simulink model "sixuanyi_test"  (R2020a)
settings: Solver=ode45  StartTime=0.0  StopTime=inf  RelTol=1e-3
values from neighbouring files (symbols this model uses):
  P =     [Pdata.mat]
undefined symbols (not defined in the file or in its folder): plot_tracjectory
libraries: simulink x4
settings Model: Creator=陈帅  LastModifiedBy=陈帅

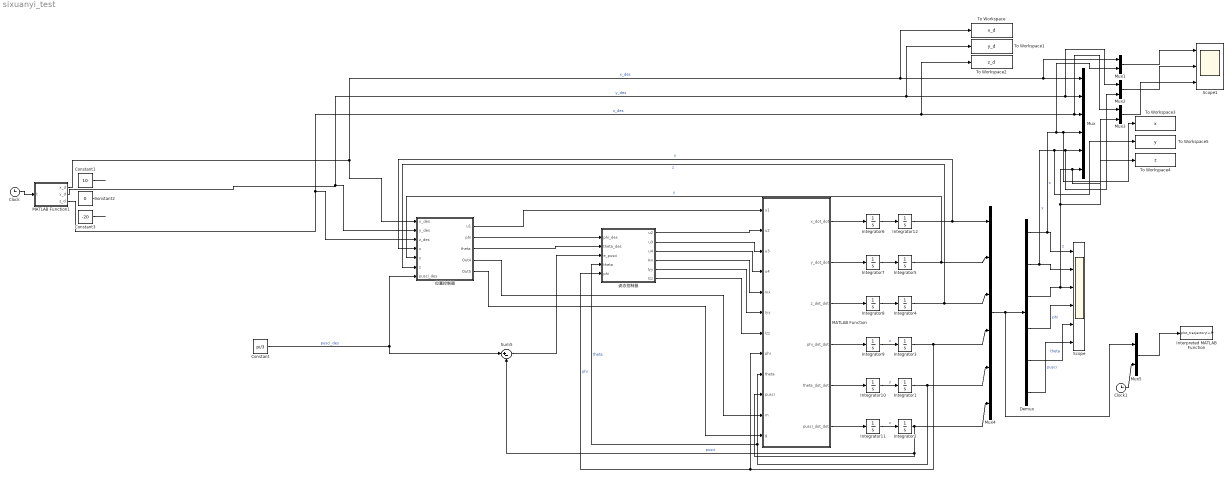
== system sixuanyi_test ==
  Clock : Clock
  Clock1 : Clock
  Constant : Constant  Value=pi/3
  Constant1 : Constant  Value=10
  Constant2 : Constant  Value=0
  Constant3 : Constant  Value=-20
  Demux : Demux  Outputs=6
  Integrator{1..12} (12 alike) : Integrator
  Interpreted MATLAB Function : MATLABFcn  MATLABFcn=plot_tracjectory(u,P)  OutputDimensions=0
  MATLAB Function : MATLAB Function  TreatAsAtomicUnit=on
  MATLAB Function1 : MATLAB Function  TreatAsAtomicUnit=on
  Mux : Mux  Inputs=6
  Mux{1..3,5} (4 alike) : Mux  Inputs=2
  Mux4 : Mux  Inputs=6
  Scope : Scope  NumInputPorts=6
  Scope1 : Scope  NumInputPorts=3
  Sum5 : Sum  Inputs=|+-
  To Workspace : ToWorkspace  VariableName=x_d  SampleTime=-1
      settings: Save2DSignal=2-D array (concatenate along first dimension)
  To Workspace1 : ToWorkspace  VariableName=y_d  SampleTime=-1
      settings: Save2DSignal=2-D array (concatenate along first dimension)
  To Workspace2 : ToWorkspace  VariableName=z_d  SampleTime=-1
      settings: Save2DSignal=2-D array (concatenate along first dimension)
  To Workspace3 : ToWorkspace  VariableName=x  SampleTime=-1
      settings: Save2DSignal=2-D array (concatenate along first dimension)
  To Workspace4 : ToWorkspace  VariableName=z  SampleTime=-1
      settings: Save2DSignal=2-D array (concatenate along first dimension)
  To Workspace5 : ToWorkspace  VariableName=y  SampleTime=-1
      settings: Save2DSignal=2-D array (concatenate along first dimension)
  位置控制器 : Subsystem
  姿态控制器 : Subsystem
  wires:
  Integrator9/1 -> Integrator3/1  "x"
  Integrator10/1 -> Integrator1/1  "y"
  Integrator11/1 -> Integrator2/1  "z"
  MATLAB Function/4(phi_dot_dot) -> Integrator9/1
  MATLAB Function/5(theta_dot_dot) -> Integrator10/1
  MATLAB Function/6(pusci_dot_dot) -> Integrator11/1
  Integrator3/1 -> 姿态控制器/5(phi), MATLAB Function/8(phi), Mux4/4  "phi"
  Integrator1/1 -> Mux4/5, 姿态控制器/4(theta), MATLAB Function/9(theta)  "theta"
  Constant/1 -> Sum5/1, 位置控制器/7(pusci_des)  "pusci_des"
  Integrator2/1 -> MATLAB Function/10(pusci), Sum5/2, Mux4/6  "pusci"
  MATLAB Function/3(z_dot_dot) -> Integrator8/1
  Integrator8/1 -> Integrator4/1
  MATLAB Function/2(y_dot_dot) -> Integrator7/1
  MATLAB Function/1(x_dot_dot) -> Integrator6/1
  Integrator6/1 -> Integrator12/1
  Integrator4/1 -> 位置控制器/6(z), Mux4/3  "z"
  Integrator7/1 -> Integrator5/1
  Integrator12/1 -> 位置控制器/4(x), Mux4/1  "x"
  Integrator5/1 -> 位置控制器/5(y), Mux4/2  "y"
  Mux4/1 -> Mux5/1, Demux/1
  Demux/1 -> Mux1/2, To Workspace3/1, Mux/4, Scope/1  "x"
  Demux/2 -> To Workspace5/1, Mux2/2, Mux/5, Scope/2  "y"
  Demux/3 -> To Workspace4/1, Mux3/2, Mux/6, Scope/3  "z"
  Demux/4 -> Scope/4  "phi"
  Demux/5 -> Scope/5  "theta"
  Demux/6 -> Scope/6  "pusci"
  Sum5/1 -> 姿态控制器/3(e_pusci)
  姿态控制器/1(u2) -> MATLAB Function/2(u2)
  姿态控制器/2(u3) -> MATLAB Function/3(u3)
  姿态控制器/3(u4) -> MATLAB Function/4(u4)
  姿态控制器/4(Ixx) -> MATLAB Function/5(Ixx)
  姿态控制器/5(Iyy) -> MATLAB Function/6(Iyy)
  姿态控制器/6(Izz) -> MATLAB Function/7(Izz)
  MATLAB Function1/1(x_d) -> 位置控制器/1(x_des), To Workspace/1, Mux1/1, Mux/1  "x_des"
  MATLAB Function1/2(y_d) -> To Workspace1/1, Mux2/1, Mux/2, 位置控制器/2(y_des)  "y_des"
  MATLAB Function1/3(z_d) -> To Workspace2/1, Mux3/1, Mux/3, 位置控制器/3(z_des)  "z_des"
  位置控制器/1(u1) -> MATLAB Function/1(u1)
  位置控制器/2(phi) -> 姿态控制器/1(phi_des)
  位置控制器/3(theta) -> 姿态控制器/2(theta_des)
  位置控制器/4(Out4) -> MATLAB Function/11(m)
  位置控制器/5(Out5) -> MATLAB Function/12(g)
  Mux1/1 -> Scope1/1
  Mux2/1 -> Scope1/2
  Mux3/1 -> Scope1/3
  Mux5/1 -> Interpreted MATLAB Function/1
  Clock1/1 -> Mux5/2
  Constant1/1 -> ?
  Constant2/1 -> ?
  Constant3/1 -> ?
  Clock/1 -> MATLAB Function1/1(t)

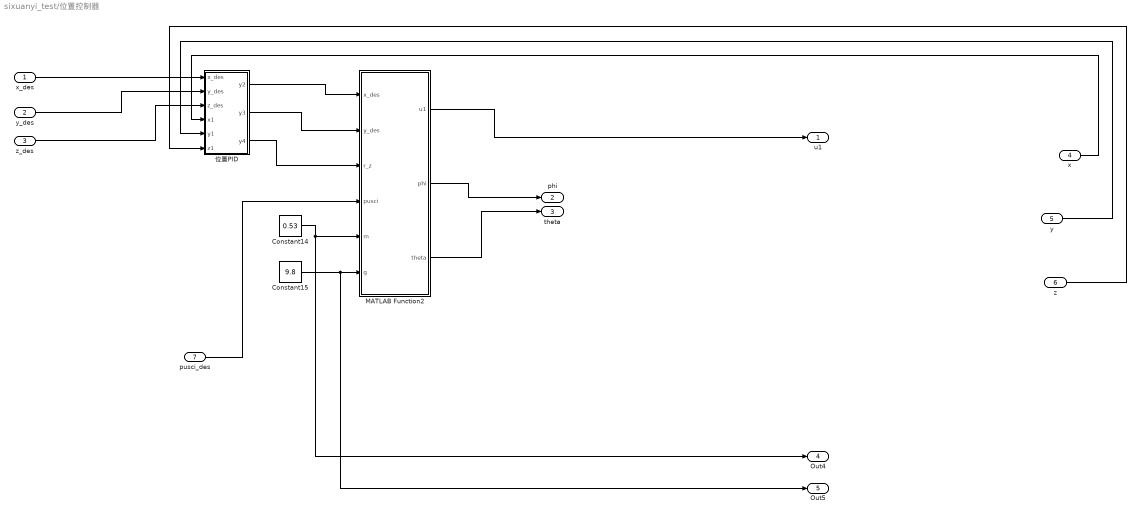
== system sixuanyi_test/位置控制器 ==
  x_des : Inport
  y_des : Inport  Port=2
  z_des : Inport  Port=3
  x : Inport  Port=4
  y : Inport  Port=5
  z : Inport  Port=6
  pusci_des : Inport  Port=7
  Constant14 : Constant  Value=0.53
  Constant15 : Constant  Value=9.8
  MATLAB Function2 : MATLAB Function  TreatAsAtomicUnit=on
  位置PID : Subsystem
  u1 : Outport
  phi : Outport  Port=2
  theta : Outport  Port=3
  Out4 : Outport  Port=4
  Out5 : Outport  Port=5
  wires:
  Constant14/1 -> Out4/1, MATLAB Function2/5(m)
  位置PID/1(y2) -> MATLAB Function2/1(x_des)
  y/1 -> 位置PID/5(y1)
  MATLAB Function2/3(theta) -> theta/1
  pusci_des/1 -> MATLAB Function2/4(pusci)
  位置PID/2(y3) -> MATLAB Function2/2(y_des)
  y_des/1 -> 位置PID/2(y_des)
  Constant15/1 -> Out5/1, MATLAB Function2/6(g)
  MATLAB Function2/1(u1) -> u1/1
  x_des/1 -> 位置PID/1(x_des)
  位置PID/3(y4) -> MATLAB Function2/3(r_z)
  x/1 -> 位置PID/4(x1)
  MATLAB Function2/2(phi) -> phi/1
  z/1 -> 位置PID/6(z1)
  z_des/1 -> 位置PID/3(z_des)

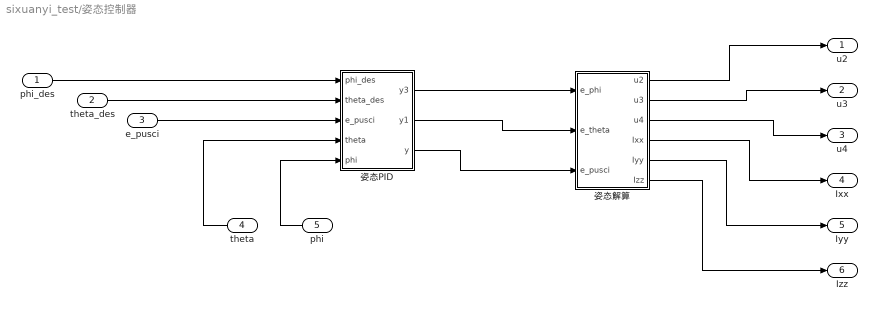
== system sixuanyi_test/姿态控制器 ==
  phi_des : Inport
  theta_des : Inport  Port=2
  e_pusci : Inport  Port=3
  theta : Inport  Port=4
  phi : Inport  Port=5
  姿态PID : Subsystem
  姿态解算 : Subsystem
  u2 : Outport
  u3 : Outport  Port=2
  u4 : Outport  Port=3
  Ixx : Outport  Port=4
  Iyy : Outport  Port=5
  Izz : Outport  Port=6
  wires:
  姿态解算/3(u4) -> u4/1
  姿态PID/2(y1) -> 姿态解算/2(e_theta)
  姿态解算/5(Iyy) -> Iyy/1
  姿态解算/6(Izz) -> Izz/1
  姿态PID/3(y) -> 姿态解算/3(e_pusci)
  姿态PID/1(y3) -> 姿态解算/1(e_phi)
  phi_des/1 -> 姿态PID/1(phi_des)
  e_pusci/1 -> 姿态PID/3(e_pusci)
  姿态解算/4(Ixx) -> Ixx/1
  姿态解算/2(u3) -> u3/1
  姿态解算/1(u2) -> u2/1
  theta_des/1 -> 姿态PID/2(theta_des)
  phi/1 -> 姿态PID/5(phi)
  theta/1 -> 姿态PID/4(theta)

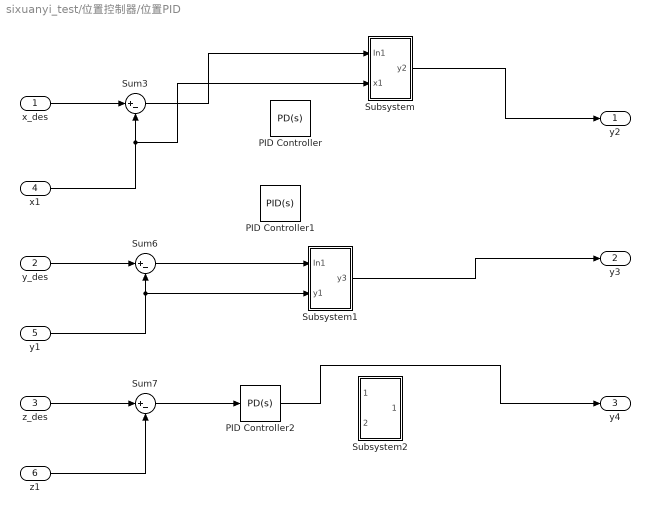
== system sixuanyi_test/位置控制器/位置PID ==
  x_des : Inport
  y_des : Inport  Port=2
  z_des : Inport  Port=3
  x1 : Inport  Port=4
  y1 : Inport  Port=5
  z1 : Inport  Port=6
  PID Controller : simulink/Continuous/PID Controller  Controller=PD  Form=Parallel  TimeDomain=Continuous-time  UseExternalTs=off  SampleTime=-1  IntegratorMethod=Forward Euler  FilterMethod=Forward Euler  ControllerParametersSource=internal  P=0.0127137328942064  I=6.25628714194927e-05  D=0.574050981950461  UseFilter=on  N=96.3969564252271  TunerSelectOption=Transfer Function Based (PID Tuner App)  InitialConditionSource=internal  InitialConditionForIntegrator=0  InitialConditionForFilter=0  DifferentiatorICPrevScaledInput=0  ExternalReset=none  TrackingMode=off  Kt=1  LimitOutput=off  UpperSaturationLimit=inf  LowerSaturationLimit=-inf  LinearizeAsGain=on  AntiWindupMode=none  Kb=1  POutMin=[]  POutMax=[]  IOutMin=[]  IOutMax=[]  DOutMin=[]  DOutMax=[]  NOutMin=[]  NOutMax=[]  SumOutMin=[]  SumOutMax=[]  SaturationOutMin=[]  SaturationOutMax=[]  PParamMin=[]  PParamMax=[]  IParamMin=[]  IParamMax=[]  DParamMin=[]  DParamMax=[]  NParamMin=[]  NParamMax=[]  KbParamMin=[]  KbParamMax=[]  KtParamMin=[]  KtParamMax=[]  KbOutMin=[]  KbOutMax=[]  KtOutMin=[]  KtOutMax=[]  IntegratorOutMin=[]  IntegratorOutMax=[]  FilterOutMin=[]  FilterOutMax=[]  SumI1OutMin=[]  SumI1OutMax=[]  SumI2OutMin=[]  SumI2OutMax=[]  SumI3OutMin=[]  SumI3OutMax=[]  SumI4OutMin=[]  SumI4OutMax=[]  SumDOutMin=[]  SumDOutMax=[]  DifferentiatorOutMin=[]  DifferentiatorOutMax=[]  FilterDiffOutCoefMin=[]  FilterDiffOutCoefMax=[]  ReciprocalOutMin=[]  ReciprocalOutMax=[]  SumDenOutMin=[]  SumDenOutMax=[]  SumNumOutMin=[]  SumNumOutMax=[]  DivideOutMin=[]  DivideOutMax=[]  UdiffTsProdOutMin=[]  UdiffTsProdOutMax=[]  NTsProdOutMin=[]  NTsProdOutMax=[]  UintegralTsProdOutMin=[]  UintegralTsProdOutMax=[]  UngainTsProdOutMin=[]  UngainTsProdOutMax=[]  IntegratorContinuousStateAttributes=''  IntegratorStateMustResolveToSignalObject=off  IntegratorRTWStateStorageClass=Auto  FilterContinuousStateAttributes=''  FilterStateMustResolveToSignalObject=off  FilterRTWStateStorageClass=Auto  ParallelPVariant=InternalParameters  IdealPVariant=Disabled  IVariant=Disabled  DVariant=InternalParameters  IntegratorVariant=Disabled  SatVariant=Disabled  AWVariant=Disabled  PCopyVariant=Disabled  TRVariant=Disabled  FdbkBlocksVariant=Forward  IdealPFdbkVariant=Disabled  SatFdbkVariant=Disabled  DerivativeFilterVariant=ContFilter  NVariant=InternalParameters  NCopyVariant=Disabled  FilterICVariant=InternalICsFilter  IntegratorICVariant=Disabled  ExternalResetVariant=Disabled  TRSumVariant=Passthrough  SumFdbkVariant=Disabled  SumVariant=Sum_PD  TsampFilterVariant=InternalTs  TsampNgainVariant=Passthrough  TsampIntegralVariant=Disabled_SignalSpec
  PID Controller1 : simulink/Continuous/PID Controller  Controller=PID  Form=Parallel  TimeDomain=Continuous-time  UseExternalTs=off  SampleTime=-1  IntegratorMethod=Forward Euler  FilterMethod=Forward Euler  ControllerParametersSource=internal  P=0.0236681294333178  I=0  D=0.611835999148078  UseFilter=on  N=102.587789590808  TunerSelectOption=Transfer Function Based (PID Tuner App)  InitialConditionSource=internal  InitialConditionForIntegrator=0  InitialConditionForFilter=0  DifferentiatorICPrevScaledInput=0  ExternalReset=none  TrackingMode=off  Kt=1  LimitOutput=off  UpperSaturationLimit=inf  LowerSaturationLimit=-inf  LinearizeAsGain=on  AntiWindupMode=none  Kb=1  POutMin=[]  POutMax=[]  IOutMin=[]  IOutMax=[]  DOutMin=[]  DOutMax=[]  NOutMin=[]  NOutMax=[]  SumOutMin=[]  SumOutMax=[]  SaturationOutMin=[]  SaturationOutMax=[]  PParamMin=[]  PParamMax=[]  IParamMin=[]  IParamMax=[]  DParamMin=[]  DParamMax=[]  NParamMin=[]  NParamMax=[]  KbParamMin=[]  KbParamMax=[]  KtParamMin=[]  KtParamMax=[]  KbOutMin=[]  KbOutMax=[]  KtOutMin=[]  KtOutMax=[]  IntegratorOutMin=[]  IntegratorOutMax=[]  FilterOutMin=[]  FilterOutMax=[]  SumI1OutMin=[]  SumI1OutMax=[]  SumI2OutMin=[]  SumI2OutMax=[]  SumI3OutMin=[]  SumI3OutMax=[]  SumI4OutMin=[]  SumI4OutMax=[]  SumDOutMin=[]  SumDOutMax=[]  DifferentiatorOutMin=[]  DifferentiatorOutMax=[]  FilterDiffOutCoefMin=[]  FilterDiffOutCoefMax=[]  ReciprocalOutMin=[]  ReciprocalOutMax=[]  SumDenOutMin=[]  SumDenOutMax=[]  SumNumOutMin=[]  SumNumOutMax=[]  DivideOutMin=[]  DivideOutMax=[]  UdiffTsProdOutMin=[]  UdiffTsProdOutMax=[]  NTsProdOutMin=[]  NTsProdOutMax=[]  UintegralTsProdOutMin=[]  UintegralTsProdOutMax=[]  UngainTsProdOutMin=[]  UngainTsProdOutMax=[]  IntegratorContinuousStateAttributes=''  IntegratorStateMustResolveToSignalObject=off  IntegratorRTWStateStorageClass=Auto  FilterContinuousStateAttributes=''  FilterStateMustResolveToSignalObject=off  FilterRTWStateStorageClass=Auto  ParallelPVariant=InternalParameters  IdealPVariant=Disabled  IVariant=InternalParameters  DVariant=InternalParameters  IntegratorVariant=Continuous  SatVariant=Disabled  AWVariant=Passthrough  PCopyVariant=Disabled  TRVariant=Disabled  FdbkBlocksVariant=Forward  IdealPFdbkVariant=Disabled  SatFdbkVariant=Disabled  DerivativeFilterVariant=ContFilter  NVariant=InternalParameters  NCopyVariant=Disabled  FilterICVariant=InternalICsFilter  IntegratorICVariant=InternalICs  ExternalResetVariant=Disabled  TRSumVariant=Passthrough  SumFdbkVariant=Disabled  SumVariant=Sum_PID  TsampFilterVariant=InternalTs  TsampNgainVariant=Passthrough  TsampIntegralVariant=Passthrough
  PID Controller2 : simulink/Continuous/PID Controller  Controller=PD  Form=Parallel  TimeDomain=Continuous-time  UseExternalTs=off  SampleTime=-1  IntegratorMethod=Forward Euler  FilterMethod=Forward Euler  ControllerParametersSource=internal  P=1.56802475831862  I=1  D=8.31416999663837  UseFilter=on  N=950.562907073993  TunerSelectOption=Transfer Function Based (PID Tuner App)  InitialConditionSource=internal  InitialConditionForIntegrator=0  InitialConditionForFilter=0  DifferentiatorICPrevScaledInput=0  ExternalReset=none  TrackingMode=off  Kt=1  LimitOutput=off  UpperSaturationLimit=inf  LowerSaturationLimit=-inf  LinearizeAsGain=on  AntiWindupMode=none  Kb=1  POutMin=[]  POutMax=[]  IOutMin=[]  IOutMax=[]  DOutMin=[]  DOutMax=[]  NOutMin=[]  NOutMax=[]  SumOutMin=[]  SumOutMax=[]  SaturationOutMin=[]  SaturationOutMax=[]  PParamMin=[]  PParamMax=[]  IParamMin=[]  IParamMax=[]  DParamMin=[]  DParamMax=[]  NParamMin=[]  NParamMax=[]  KbParamMin=[]  KbParamMax=[]  KtParamMin=[]  KtParamMax=[]  KbOutMin=[]  KbOutMax=[]  KtOutMin=[]  KtOutMax=[]  IntegratorOutMin=[]  IntegratorOutMax=[]  FilterOutMin=[]  FilterOutMax=[]  SumI1OutMin=[]  SumI1OutMax=[]  SumI2OutMin=[]  SumI2OutMax=[]  SumI3OutMin=[]  SumI3OutMax=[]  SumI4OutMin=[]  SumI4OutMax=[]  SumDOutMin=[]  SumDOutMax=[]  DifferentiatorOutMin=[]  DifferentiatorOutMax=[]  FilterDiffOutCoefMin=[]  FilterDiffOutCoefMax=[]  ReciprocalOutMin=[]  ReciprocalOutMax=[]  SumDenOutMin=[]  SumDenOutMax=[]  SumNumOutMin=[]  SumNumOutMax=[]  DivideOutMin=[]  DivideOutMax=[]  UdiffTsProdOutMin=[]  UdiffTsProdOutMax=[]  NTsProdOutMin=[]  NTsProdOutMax=[]  UintegralTsProdOutMin=[]  UintegralTsProdOutMax=[]  UngainTsProdOutMin=[]  UngainTsProdOutMax=[]  IntegratorContinuousStateAttributes=''  IntegratorStateMustResolveToSignalObject=off  IntegratorRTWStateStorageClass=Auto  FilterContinuousStateAttributes=''  FilterStateMustResolveToSignalObject=off  FilterRTWStateStorageClass=Auto  ParallelPVariant=InternalParameters  IdealPVariant=Disabled  IVariant=Disabled  DVariant=InternalParameters  IntegratorVariant=Disabled  SatVariant=Disabled  AWVariant=Disabled  PCopyVariant=Disabled  TRVariant=Disabled  FdbkBlocksVariant=Forward  IdealPFdbkVariant=Disabled  SatFdbkVariant=Disabled  DerivativeFilterVariant=ContFilter  NVariant=InternalParameters  NCopyVariant=Disabled  FilterICVariant=InternalICsFilter  IntegratorICVariant=Disabled  ExternalResetVariant=Disabled  TRSumVariant=Passthrough  SumFdbkVariant=Disabled  SumVariant=Sum_PD  TsampFilterVariant=InternalTs  TsampNgainVariant=Passthrough  TsampIntegralVariant=Disabled_SignalSpec
  Subsystem : Subsystem
  Subsystem1 : Subsystem
  Subsystem2 : Subsystem
  Sum3 : Sum  Inputs=|+-
  Sum6 : Sum  Inputs=|+-
  Sum7 : Sum  Inputs=|+-
  y2 : Outport
  y3 : Outport  Port=2
  y4 : Outport  Port=3
  wires:
  z_des/1 -> Sum7/1
  y_des/1 -> Sum6/1
  x1/1 -> Subsystem/2(x1), Sum3/2
  x_des/1 -> Sum3/1
  y1/1 -> Subsystem1/2(y1), Sum6/2
  z1/1 -> Sum7/2
  Sum7/1 -> PID Controller2/1
  PID Controller2/1 -> y4/1
  Subsystem1/1(y3) -> y3/1
  Sum6/1 -> Subsystem1/1(In1)
  Sum3/1 -> Subsystem/1(In1)
  Subsystem/1(y2) -> y2/1

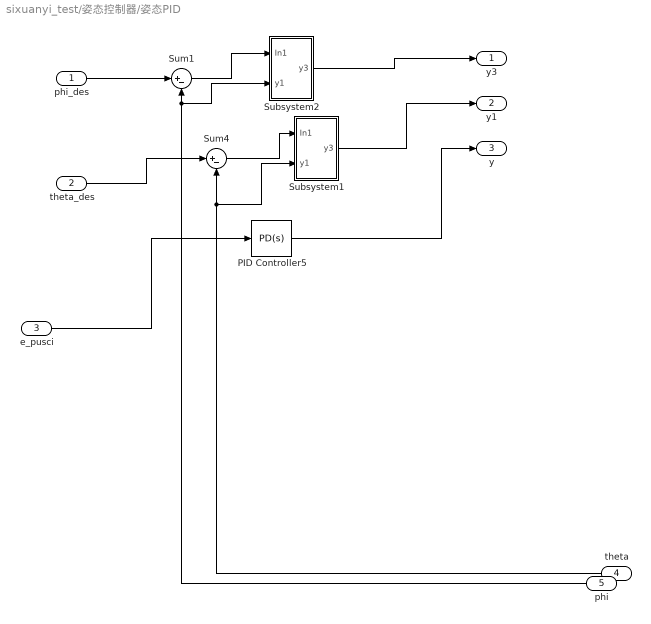
== system sixuanyi_test/姿态控制器/姿态PID ==
  phi_des : Inport
  theta_des : Inport  Port=2
  e_pusci : Inport  Port=3
  theta : Inport  Port=4
  phi : Inport  Port=5
  PID Controller5 : simulink/Continuous/PID Controller  Controller=PD  Form=Parallel  TimeDomain=Continuous-time  UseExternalTs=off  SampleTime=-1  IntegratorMethod=Forward Euler  FilterMethod=Forward Euler  ControllerParametersSource=internal  P=5.26569653292964  I=0  D=4.89151407738421  UseFilter=on  N=572.770791824144  TunerSelectOption=Transfer Function Based (PID Tuner App)  InitialConditionSource=internal  InitialConditionForIntegrator=0  InitialConditionForFilter=0  DifferentiatorICPrevScaledInput=0  ExternalReset=none  TrackingMode=off  Kt=1  LimitOutput=off  UpperSaturationLimit=inf  LowerSaturationLimit=-inf  LinearizeAsGain=on  AntiWindupMode=none  Kb=1  POutMin=[]  POutMax=[]  IOutMin=[]  IOutMax=[]  DOutMin=[]  DOutMax=[]  NOutMin=[]  NOutMax=[]  SumOutMin=[]  SumOutMax=[]  SaturationOutMin=[]  SaturationOutMax=[]  PParamMin=[]  PParamMax=[]  IParamMin=[]  IParamMax=[]  DParamMin=[]  DParamMax=[]  NParamMin=[]  NParamMax=[]  KbParamMin=[]  KbParamMax=[]  KtParamMin=[]  KtParamMax=[]  KbOutMin=[]  KbOutMax=[]  KtOutMin=[]  KtOutMax=[]  IntegratorOutMin=[]  IntegratorOutMax=[]  FilterOutMin=[]  FilterOutMax=[]  SumI1OutMin=[]  SumI1OutMax=[]  SumI2OutMin=[]  SumI2OutMax=[]  SumI3OutMin=[]  SumI3OutMax=[]  SumI4OutMin=[]  SumI4OutMax=[]  SumDOutMin=[]  SumDOutMax=[]  DifferentiatorOutMin=[]  DifferentiatorOutMax=[]  FilterDiffOutCoefMin=[]  FilterDiffOutCoefMax=[]  ReciprocalOutMin=[]  ReciprocalOutMax=[]  SumDenOutMin=[]  SumDenOutMax=[]  SumNumOutMin=[]  SumNumOutMax=[]  DivideOutMin=[]  DivideOutMax=[]  UdiffTsProdOutMin=[]  UdiffTsProdOutMax=[]  NTsProdOutMin=[]  NTsProdOutMax=[]  UintegralTsProdOutMin=[]  UintegralTsProdOutMax=[]  UngainTsProdOutMin=[]  UngainTsProdOutMax=[]  IntegratorContinuousStateAttributes=''  IntegratorStateMustResolveToSignalObject=off  IntegratorRTWStateStorageClass=Auto  FilterContinuousStateAttributes=''  FilterStateMustResolveToSignalObject=off  FilterRTWStateStorageClass=Auto  ParallelPVariant=InternalParameters  IdealPVariant=Disabled  IVariant=Disabled  DVariant=InternalParameters  IntegratorVariant=Disabled  SatVariant=Disabled  AWVariant=Disabled  PCopyVariant=Disabled  TRVariant=Disabled  FdbkBlocksVariant=Forward  IdealPFdbkVariant=Disabled  SatFdbkVariant=Disabled  DerivativeFilterVariant=ContFilter  NVariant=InternalParameters  NCopyVariant=Disabled  FilterICVariant=InternalICsFilter  IntegratorICVariant=Disabled  ExternalResetVariant=Disabled  TRSumVariant=Passthrough  SumFdbkVariant=Disabled  SumVariant=Sum_PD  TsampFilterVariant=InternalTs  TsampNgainVariant=Passthrough  TsampIntegralVariant=Disabled_SignalSpec
  Subsystem1 : Subsystem
  Subsystem2 : Subsystem
  Sum1 : Sum  Inputs=|+-
  Sum4 : Sum  Inputs=|+-
  y3 : Outport
  y1 : Outport  Port=2
  y : Outport  Port=3
  wires:
  Sum4/1 -> Subsystem1/1(In1)
  theta_des/1 -> Sum4/1
  phi_des/1 -> Sum1/1
  theta/1 -> Subsystem1/2(y1), Sum4/2
  phi/1 -> Subsystem2/2(y1), Sum1/2
  PID Controller5/1 -> y/1
  e_pusci/1 -> PID Controller5/1
  Subsystem2/1(y3) -> y3/1
  Sum1/1 -> Subsystem2/1(In1)
  Subsystem1/1(y3) -> y1/1

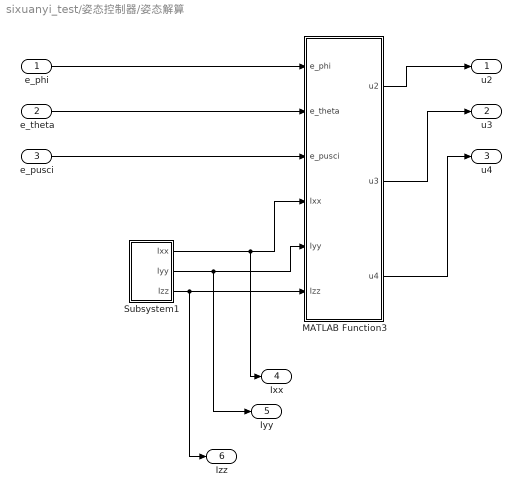
== system sixuanyi_test/姿态控制器/姿态解算 ==
  e_phi : Inport
  e_theta : Inport  Port=2
  e_pusci : Inport  Port=3
  MATLAB Function3 : MATLAB Function  TreatAsAtomicUnit=on
  Subsystem1 : Subsystem
  u2 : Outport
  u3 : Outport  Port=2
  u4 : Outport  Port=3
  Ixx : Outport  Port=4
  Iyy : Outport  Port=5
  Izz : Outport  Port=6
  wires:
  e_theta/1 -> MATLAB Function3/2(e_theta)
  Subsystem1/2(Iyy) -> MATLAB Function3/5(Iyy), Iyy/1
  Subsystem1/1(Ixx) -> MATLAB Function3/4(Ixx), Ixx/1
  e_pusci/1 -> MATLAB Function3/3(e_pusci)
  Subsystem1/3(Izz) -> MATLAB Function3/6(Izz), Izz/1
  MATLAB Function3/1(u2) -> u2/1
  e_phi/1 -> MATLAB Function3/1(e_phi)
  MATLAB Function3/2(u3) -> u3/1
  MATLAB Function3/3(u4) -> u4/1

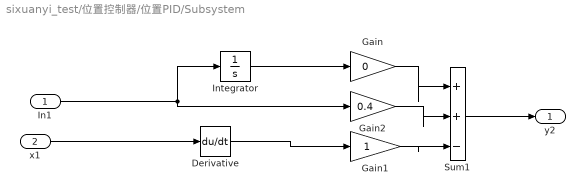
== system sixuanyi_test/位置控制器/位置PID/Subsystem ==
  In1 : Inport
  x1 : Inport  Port=2
  Derivative : Derivative
  Gain : Gain  Gain=0
  Gain1 : Gain
  Gain2 : Gain  Gain=0.4
  Integrator : Integrator
  Sum1 : Sum  Inputs=|++-
  y2 : Outport
  wires:
  In1/1 -> Gain2/1, Integrator/1
  Gain/1 -> Sum1/1
  Derivative/1 -> Gain1/1
  Gain1/1 -> Sum1/3
  Integrator/1 -> Gain/1
  Sum1/1 -> y2/1
  Gain2/1 -> Sum1/2
  x1/1 -> Derivative/1

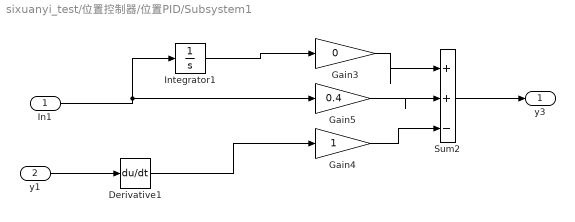
== system sixuanyi_test/位置控制器/位置PID/Subsystem1 ==
  In1 : Inport
  y1 : Inport  Port=2
  Derivative1 : Derivative
  Gain3 : Gain  Gain=0
  Gain4 : Gain
  Gain5 : Gain  Gain=0.4
  Integrator1 : Integrator
  Sum2 : Sum  Inputs=|++-
  y3 : Outport
  wires:
  Integrator1/1 -> Gain3/1
  In1/1 -> Integrator1/1, Gain5/1
  Gain4/1 -> Sum2/3
  Derivative1/1 -> Gain4/1
  Gain3/1 -> Sum2/1
  y1/1 -> Derivative1/1
  Gain5/1 -> Sum2/2
  Sum2/1 -> y3/1

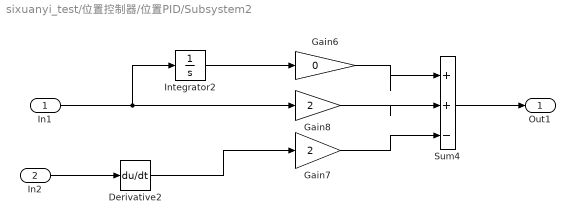
== system sixuanyi_test/位置控制器/位置PID/Subsystem2 ==
  In1 : Inport
  In2 : Inport  Port=2
  Derivative2 : Derivative
  Gain6 : Gain  Gain=0
  Gain7 : Gain  Gain=2
  Gain8 : Gain  Gain=2
  Integrator2 : Integrator
  Sum4 : Sum  Inputs=|++-
  Out1 : Outport
  wires:
  In2/1 -> Derivative2/1
  Integrator2/1 -> Gain6/1
  Gain6/1 -> Sum4/1
  Derivative2/1 -> Gain7/1
  Gain8/1 -> Sum4/2
  Gain7/1 -> Sum4/3
  In1/1 -> Integrator2/1, Gain8/1
  Sum4/1 -> Out1/1

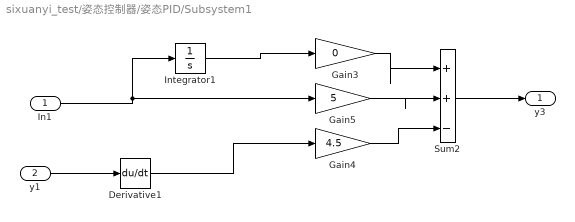
== system sixuanyi_test/姿态控制器/姿态PID/Subsystem1 ==
  In1 : Inport
  y1 : Inport  Port=2
  Derivative1 : Derivative
  Gain3 : Gain  Gain=0
  Gain4 : Gain  Gain=4.5
  Gain5 : Gain  Gain=5
  Integrator1 : Integrator
  Sum2 : Sum  Inputs=|++-
  y3 : Outport
  wires:
  Integrator1/1 -> Gain3/1
  In1/1 -> Integrator1/1, Gain5/1
  Gain4/1 -> Sum2/3
  Derivative1/1 -> Gain4/1
  Gain3/1 -> Sum2/1
  y1/1 -> Derivative1/1
  Gain5/1 -> Sum2/2
  Sum2/1 -> y3/1

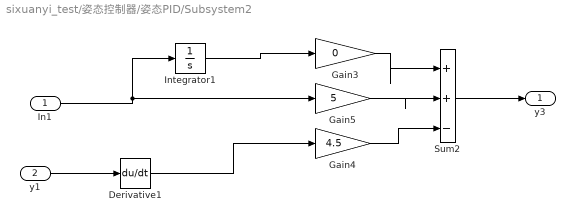
== system sixuanyi_test/姿态控制器/姿态PID/Subsystem2 ==
  In1 : Inport
  y1 : Inport  Port=2
  Derivative1 : Derivative
  Gain3 : Gain  Gain=0
  Gain4 : Gain  Gain=4.5
  Gain5 : Gain  Gain=5
  Integrator1 : Integrator
  Sum2 : Sum  Inputs=|++-
  y3 : Outport
  wires:
  Sum2/1 -> y3/1
  Gain5/1 -> Sum2/2
  y1/1 -> Derivative1/1
  Gain3/1 -> Sum2/1
  Derivative1/1 -> Gain4/1
  Gain4/1 -> Sum2/3
  In1/1 -> Gain5/1, Integrator1/1
  Integrator1/1 -> Gain3/1

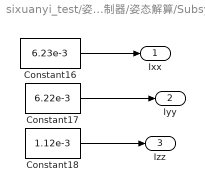
== system sixuanyi_test/姿态控制器/姿态解算/Subsystem1 ==
  Constant16 : Constant  Value=6.23e-3
  Constant17 : Constant  Value=6.22e-3
  Constant18 : Constant  Value=1.12e-3
  Ixx : Outport
  Iyy : Outport  Port=2
  Izz : Outport  Port=3
  wires:
  Constant18/1 -> Izz/1
  Constant16/1 -> Ixx/1
  Constant17/1 -> Iyy/1

== matlab function sixuanyi_test/MATLAB Function1 ==
  data: t input; x_d output; y_d output; z_d output
function [x_d,y_d,z_d]= fcn(t)
x_d=cos(t/2);
y_d=sin(t/2);
z_d=-0.2*t;
end

== matlab function sixuanyi_test/MATLAB Function ==
  data: u1 input; u2 input; u3 input; u4 input; x_dot_dot output; y_dot_dot output; z_dot_dot output; phi_dot_dot output; theta_dot_dot output; pusci_dot_dot output; Ixx input; Iyy input; Izz input; phi input; theta input; pusci input; m input; g input
function [x_dot_dot,y_dot_dot,z_dot_dot,phi_dot_dot,theta_dot_dot,pusci_dot_dot]=dynamic(u1,u2,u3,u4,Ixx,Iyy,Izz,phi,theta,pusci,m,g)

x_dot_dot=-u1/m*(sin(pusci)*phi+cos(pusci)*theta);
y_dot_dot=-u1/m*(-cos(pusci)*phi+theta*sin(pusci));
z_dot_dot=g-u1/m*cos(theta)*cos(phi);

phi_dot_dot=u2/Ixx;
theta_dot_dot=u3/Iyy;
pusci_dot_dot=u4/Izz;

end

== matlab function sixuanyi_test/位置控制器/MATLAB Function2 ==
  data: u1 output; x_des input; y_des input; r_z input; pusci input; m input; g input; phi output; theta output
function [u1,phi,theta]=position_controller(x_des,y_des, r_z,pusci,m,g)

u1=(g-r_z)*m;
R=[
cos(pusci),-sin(pusci);
sin(pusci),cos(pusci)
];
A=[
    sin(pusci),cos(pusci);
    -cos(pusci),sin(pusci)
    ];
r_des=[x_des;y_des];
tempt=-1/g*inv(A)*r_des;
phi=tempt(1);
theta=tempt(2);



end

== matlab function sixuanyi_test/姿态控制器/姿态解算/MATLAB Function3 ==
  data: e_phi input; u2 output; e_theta input; e_pusci input; Ixx input; Iyy input; Izz input; u3 output; u4 output
function [u2,u3,u4] = attitude_controller(e_phi,e_theta,e_pusci,Ixx,Iyy,Izz)

u2=Ixx*e_phi;
u3=Iyy*e_theta;
u4=Izz*e_pusci;

end
